simulink model "Valenton_JJ_Simulink_No7"  (R2023b)
settings: Solver=VariableStepAuto  StartTime=0.0  StopTime=20  RelTol=1e-3
values from neighbouring files (symbols this model uses):
  G_den = [M B k]    [Valenton_JJ_MATLAB_No2.m]    (also in Valenton_JJ_MATLAB_No7.m = [f g h i j k])
  G_num = [1]    [Valenton_JJ_MATLAB_No2.m]    (also in Valenton_JJ_MATLAB_No7.m = [a b c d e])
settings Model: Creator=jezryl james  LastModifiedBy=jezryl james

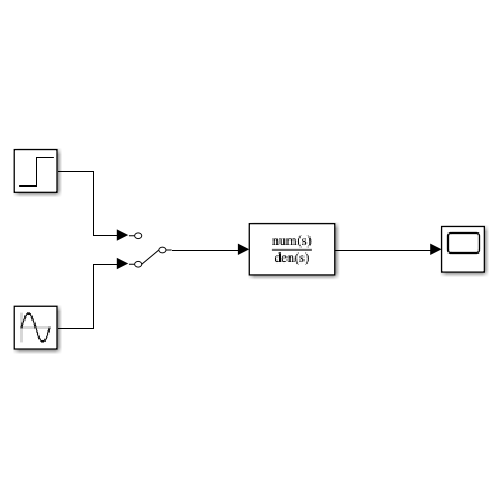
[thumbnail: Simulink's stored preview of the top-level diagram]
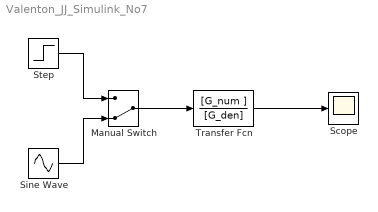
== system Valenton_JJ_Simulink_No7 ==
  Manual Switch : ManualSwitch  CurrentSetting=0
  Scope : Scope
  Sine Wave : Sin  SampleTime=0
  Step : Step  Time=0  After=0  SampleTime=0
  Transfer Fcn : TransferFcn  Numerator=[G_num ]  Denominator=[G_den]  ParameterTunability=Optimized
  wires:
  Transfer Fcn/1 -> Scope/1
  Step/1 -> Manual Switch/1
  Sine Wave/1 -> Manual Switch/2
  Manual Switch/1 -> Transfer Fcn/1
